simulink model "Einmassenschwinger"  (R2020b)
settings: Solver=ode45  StartTime=0.0  StopTime=100  RelTol=1e-6  AbsTol=1e-6  EnableMultiTasking=on
undefined symbols (not defined in the file or in its folder): parSim
libraries: cstblocks x3, simulink x2
settings Model: Creator=tg  LastModifiedBy=paul
settings SolverCC: AutoScaleAbsTol=off
settings DataIOCC: LimitDataPoints=on  SaveFormat=Array  SignalLoggingSaveFormat=ModelDataLogs  ReturnWorkspaceOutputs=off
settings OptimizationCC: ExpressionDepthLimit=2147483647  InitFltsAndDblsToZero=on  LifeSpan=inf
settings DebuggingCC: UnderspecifiedInitializationDetection=Classic  MergeDetectMultiDrivingBlocksExec=none  SolverPrmCheckMsg=warning  FcnCallInpInsideContextMsg=warning  StateNameClashWarn=warning  SFUnexpectedBacktrackingDiag=warning  SFNoUnconditionalDefaultTransitionDiag=warning  SFExecutionAtInitializationDiag=none  ArithmeticOperatorsInVariantConditions=warning
settings HardwareCC: ProdBitPerPointer=32  ProdBitPerSizeT=32  ProdBitPerPtrDiffT=32  ProdLargestAtomicFloat=None  ProdIntDivRoundTo=Undefined  ProdEndianess=Unspecified  ProdWordSize=32  ProdHWDeviceType=32-bit Generic
settings ModelReferenceCC: PropagateSignalLabelsOutOfModel=off
settings SFSimCC: SimUseLocalCustomCode=off  SimParseCustomCode=off  CustomCodeUndefinedFunction=UseInterfaceOnly
settings RTWCC: RTWUseLocalCustomCode=off
settings CodeAppCC: StateflowObjectComments=on
settings GRTTargetCC: TargetLangStandard=C89/C90 (ANSI)  CombineOutputUpdateFcns=off  GRTInterface=on
settings ConfigComp: CovMetricSettings=dw  CovSaveCumulativeToWorkspaceVar=on  CovSaveSingleToWorkspaceVar=on  CovExternalEMLEnable=off

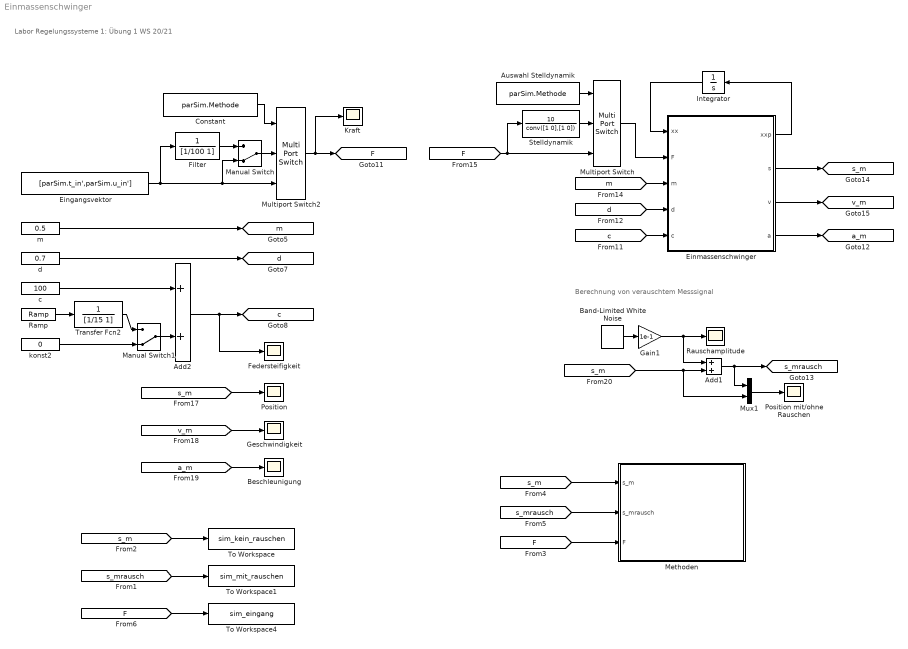
== system Einmassenschwinger ==
  note: Labor Regelungssysteme 1: Übung 1
      | WS 20/21
  note: Berechnung von verauschtem Messsignal
  Add1 : Sum
  Add2 : Sum
  Auswahl Stelldynamik : Constant  Value=parSim.Methode
  Band-Limited White Noise : simulink/Sources/Band-Limited White Noise  Cov=[1e-6]  Ts=1e-3  seed=[24341]
  Beschleunigung : Scope
  Constant : Constant  Value=parSim.Methode
  Eingangsvektor : FromWorkspace  VariableName=[parSim.t_in',parSim.u_in']  SampleTime=parSim.T_a
  Einmassenschwinger : MATLAB Function  TreatAsAtomicUnit=on
  Federsteifigkeit : Scope
  Filter : TransferFcn  Denominator=[1/100 1]
  Gain1 : Gain  Gain=1e-1
  Geschwindigkeit : Scope
  Integrator : Integrator  InitialCondition=parSim.xx0'
  Kraft : Scope
  Manual Switch : ManualSwitch  CurrentSetting=0
  Manual Switch1 : ManualSwitch  CurrentSetting=0
  Methoden : Subsystem  Variant=on  AllowZeroVariantControls=on
  Multiport Switch : MultiPortSwitch  DataPortOrder=Specify indices  Inputs=2  DataPortIndices={3,0}  DiagnosticForDefault=None
  Multiport Switch2 : MultiPortSwitch  DataPortOrder=Specify indices  Inputs=2  DataPortIndices={2,0}  DiagnosticForDefault=None
  Mux1 : Mux  Inputs=2
  Position : Scope
  Position mit/ohne Rauschen : Scope
  Ramp : simulink/Sources/Ramp  slope=0.5  start=3  InitialOutput=0
  Rauschamplitude : Scope
  Stelldynamik : TransferFcn  Numerator=[10]  Denominator=conv([1 0],[1 0])
  To Workspace : ToWorkspace  VariableName=sim_kein_rauschen  SaveFormat=Structure With Time  SampleTime=parSim.T_a
  To Workspace1 : ToWorkspace  VariableName=sim_mit_rauschen  SaveFormat=Structure With Time  SampleTime=parSim.T_a
  To Workspace4 : ToWorkspace  VariableName=sim_eingang  SaveFormat=Structure With Time  SampleTime=parSim.T_a
  Transfer Fcn2 : TransferFcn  Denominator=[1/15 1]
  c : Constant  Value=100
  d : Constant  Value=0.7
  konst2 : Constant  Value=0
  m : Constant  Value=0.5
  tag scope: F=global, a_m=global, c=global, d=global, m=global, s_m=global, s_mrausch=global, v_m=global
  wires:
  Einmassenschwinger/4(a) -> [a_m]
  d/1 -> [d]
  c/1 -> Add2/1
  Integrator/1 -> Einmassenschwinger/1(xx)
  [s_m] -> Position/1
  konst2/1 -> Manual Switch1/2
  [v_m] -> Geschwindigkeit/1
  Transfer Fcn2/1 -> Manual Switch1/1
  Einmassenschwinger/2(s) -> [s_m]
  Manual Switch1/1 -> Add2/2
  Add2/1 -> [c], Federsteifigkeit/1
  m/1 -> [m]
  [a_m] -> Beschleunigung/1
  [d] -> Einmassenschwinger/4(d)
  [m] -> Einmassenschwinger/3(m)
  [s_m] -> Add1/2, Mux1/2
  Mux1/1 -> Position mit/ohne Rauschen/1
  Ramp/1 -> Transfer Fcn2/1
  Einmassenschwinger/3(v) -> [v_m]
  Einmassenschwinger/1(xxp) -> Integrator/1
  Gain1/1 -> Rauschamplitude/1, Add1/1
  Band-Limited White Noise/1 -> Gain1/1
  [c] -> Einmassenschwinger/5(c)
  Add1/1 -> [s_mrausch], Mux1/1
  Multiport Switch/1 -> Einmassenschwinger/2(F)
  [F] -> Stelldynamik/1, Multiport Switch/3
  Auswahl Stelldynamik/1 -> Multiport Switch/1
  [F] -> To Workspace4/1
  [s_mrausch] -> To Workspace1/1
  [s_m] -> To Workspace/1
  Eingangsvektor/1 -> Manual Switch/2, Multiport Switch2/3, Filter/1
  Filter/1 -> Manual Switch/1
  Multiport Switch2/1 -> [F], Kraft/1
  [s_m] -> Methoden/1(s_m)
  [s_mrausch] -> Methoden/2(s_mrausch)
  [F] -> Methoden/3(F)
  Stelldynamik/1 -> Multiport Switch/2
  Constant/1 -> Multiport Switch2/1
  Manual Switch/1 -> Multiport Switch2/2

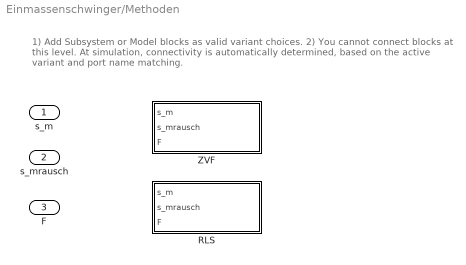
== system Einmassenschwinger/Methoden ==
  note: 1) Add Subsystem or Model blocks as valid variant choices.
      | 2) You cannot connect blocks at this level. At simulation, connectivity is automatically
      | determined, based on the active variant and port name matching.
  s_m : Inport
  s_mrausch : Inport  Port=2
  F : Inport  Port=3
  RLS : Subsystem  VariantControl=parSim.Methode == 2
  ZVF : Subsystem  VariantControl=parSim.Methode == 1

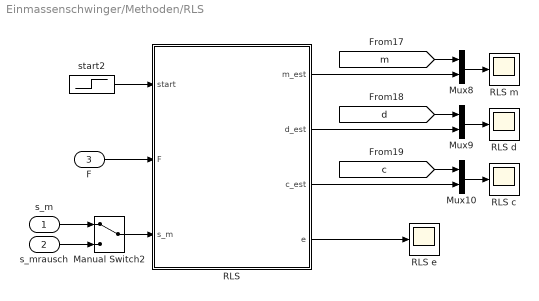
== system Einmassenschwinger/Methoden/RLS ==
  s_m : Inport
  s_mrausch : Inport  Port=2
  F : Inport  Port=3
  Manual Switch2 : ManualSwitch
  Mux10 : Mux  Inputs=2
  Mux8 : Mux  Inputs=2
  Mux9 : Mux  Inputs=2
  RLS : MATLAB Function  TreatAsAtomicUnit=on
  RLS c : Scope
  RLS d : Scope
  RLS e : Scope
  RLS m : Scope
  start2 : Step  Time=0.1  SampleTime=0
  wires:
  F/1 -> RLS/2(F)
  start2/1 -> RLS/1(start)
  RLS/1(m_est) -> Mux8/2
  RLS/4(e) -> RLS e/1
  Mux9/1 -> RLS d/1
  [d] -> Mux9/1
  s_m/1 -> Manual Switch2/1
  s_mrausch/1 -> Manual Switch2/2
  RLS/3(c_est) -> Mux10/2
  [c] -> Mux10/1
  Manual Switch2/1 -> RLS/3(s_m)
  Mux10/1 -> RLS c/1
  [m] -> Mux8/1
  RLS/2(d_est) -> Mux9/2
  Mux8/1 -> RLS m/1

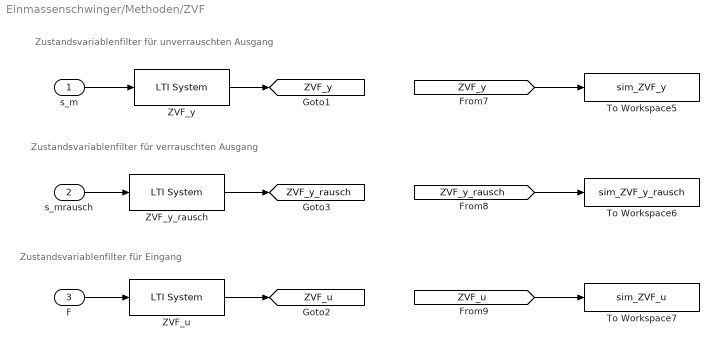
== system Einmassenschwinger/Methoden/ZVF ==
  note: Zustandsvariablenfilter für unverrauschten Ausgang
  note: Zustandsvariablenfilter für Eingang
  note: Zustandsvariablenfilter für verrauschten Ausgang
  s_m : Inport
  s_mrausch : Inport  Port=2
  F : Inport  Port=3
  To Workspace5 : ToWorkspace  VariableName=sim_ZVF_y  SaveFormat=Structure With Time  SampleTime=parSim.T_a
  To Workspace6 : ToWorkspace  VariableName=sim_ZVF_y_rausch  SaveFormat=Structure With Time  SampleTime=parSim.T_a
  To Workspace7 : ToWorkspace  VariableName=sim_ZVF_u  SaveFormat=Structure With Time  SampleTime=parSim.T_a
  ZVF_u : cstblocks/LTI System  sys=ZVFz  IC=[]
  ZVF_y : cstblocks/LTI System  sys=ZVFz  IC=[]
  ZVF_y_rausch : cstblocks/LTI System  sys=ZVFz  IC=[]
  tag scope: ZVF_u=global, ZVF_y=global, ZVF_y_rausch=global
  wires:
  F/1 -> ZVF_u/1
  ZVF_u/1 -> [ZVF_u]
  ZVF_y_rausch/1 -> [ZVF_y_rausch]
  s_m/1 -> ZVF_y/1
  s_mrausch/1 -> ZVF_y_rausch/1
  ZVF_y/1 -> [ZVF_y]
  [ZVF_u] -> To Workspace7/1
  [ZVF_y] -> To Workspace5/1
  [ZVF_y_rausch] -> To Workspace6/1

== matlab function Einmassenschwinger/Einmassenschwinger ==
  data: xx input; xxp output; F input; m input; d input; c input; s output; v output; a output
function [xxp, s, v, a] = Einmassenschwinger(xx, F, m, d ,c)
%%%%%%%%%%%%%%%%%%%%%%%%%%%%%%%%%%%%%%%%%%%%%%%%%%%%%%%%%%%%%%%%%%%%%%%%%%%
%
% Labor Regelungssysteme 1 Übung 1 - Einmassenschwinger
%
% Eingänge: xx              Zustandsvektor mit:
%             s [m]         Position
%             w [m/s]       Geschwindigkeit
%           F   [N]         Kraft
%           m   [kg]        Masse
%           d   [Ns/m]      Dämpfung
%           c   [N/m]       Federsteifigkeit
%
% Ausgänge: xxp [m]         Position
%           v... [m/s]      Geschwindigkeit
%           a... [m/s^2]    Beschleunigung
%
% Autor:        24.09.2020 | R. Lenz
% Änderungen:   
%
%%%%%%%%%%%%%%%%%%%%%%%%%%%%%%%%%%%%%%%%%%%%%%%%%%%%%%%%%%%%%%%%%%%%%%%%%%%

s = xx(1);
v = xx(2);
a = 1/m*(-d*v-c*s+F);

% Differentialgleichung
xxp = [v; a];

== matlab function Einmassenschwinger/Methoden/RLS/RLS ==
  settings: updateMethod=DISCRETE  sampleTime=parRLS.T_a
  data: start input; m_est output; F input; s_m input; parRLS parameter; d_est output; c_est output; e output
%%%%%%%%%%%%%%%%%%%%%%%%%%%%%%%%%%%%%%%%%%%%%%%%%%%%%%%%%%%%%%%%%%%%%%%%%%%
%
% Vorlage einer embedded Matlab-function für RLS 
%
% bearbeitet: 2010/11/29 Thomas König
% Änderungen: 04.10.2011 | W. Kemmetmüller
%             28.09.2020 | R. Lenz
%%%%%%%%%%%%%%%%%%%%%%%%%%%%%%%%%%%%%%%%%%%%%%%%%%%%%%%%%%%%%%%%%%%%%%%%%%%

function [m_est,d_est,c_est,e] = RLS(start, F, s_m, parRLS)

    % Parameter
    T_a = parRLS.T_a;       % Abtastzeit
    q = parRLS.q;           % Gedächtnisfaktor
    alpha = parRLS.alpha;   % Startwert Kovarianzmatrix

    persistent p_1 p_2 p_3                      % Parameter
    persistent P_11 P_12 P_13 P_22 P_23 P_33    % Kovarianzmatrix, P ist symmetrisch
    
    persistent uk uk1 uk2 yk yk1 yk2 P p_est
    if isempty(P_11) 
        % Anfangsbedingung
        p_1 = 0;
        p_2 = 0;
        p_3 = 0;

        p_est=[p_1;p_2;p_3];

        % Wähle Startwert der Kovarianzmatrix P_0 = alpha*E
        P_11 = alpha;
        P_12 = 0;
        P_13 = 0;
        P_22 = alpha;
        P_23 = 0;
        P_33 = alpha;

        P=[P_11,P_12,P_13;P_12,P_22,P_23;P_13,P_23,P_33]; %P ist symetrisch

        uk=0;
        uk1=0;
        uk2=0;

        yk=0;
        yk1=0;
        yk2=0;
        
        m_est = 0;
        d_est = 0;
        c_est = 0;
        e=0;

    else

        %Eingang schieben
        uk2=uk1;
        uk1=uk;
        uk=F;

        %Ausgang schieben
        yk2=yk1;
        yk1=yk;
        yk= s_m;

        if start

            uk_quer = uk +2 * uk1 + uk2;

            s = [-yk1; -yk2; uk_quer];
            sT = s';

            k = (P*s) / (q + sT*P*s);
            P= (P-k*sT*P)/q; 

            p_est=p_est + k * (yk-sT*p_est);


            m_est = (-1/16)*T_a^2*(p_est(1)-p_est(2)-1)/p_est(3);
            d_est = (-1/4)*T_a*(p_est(2)-1)/p_est(3);
            c_est = (1/4)*(p_est(1) + p_est(2) +1)/p_est(3);
            e = yk - sT*p_est;


        else

            m_est = 0;
            d_est = 0;
            c_est = 0;
            e=0;

        end
    end
end
